simulink model "kinematic_model"  (R2022b)
settings: Solver=FixedStepAuto  StartTime=0.0  StopTime=24  FixedStep=0.1  RelTol=1e-3
settings Model: Creator=Rajgir  LastModifiedBy=rajgir
settings DebuggingCC: UnconnectedInputMsg=warning  UnconnectedOutputMsg=warning  UnconnectedLineMsg=warning
settings ModelReferenceCC: EnableRefExpFcnMdlSchedulingChecks=on
settings RTWCC: DLArmComputeVersion=19.05

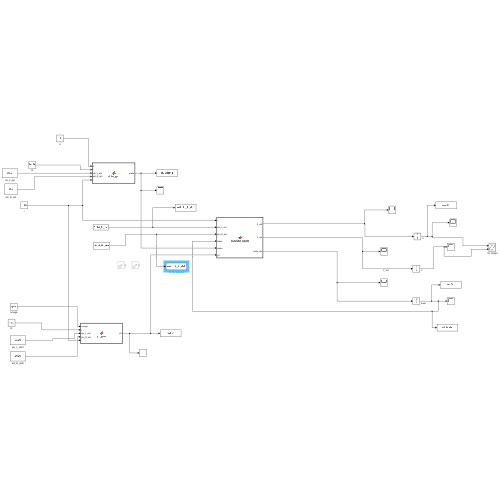
[thumbnail: Simulink's stored preview of the top-level diagram]
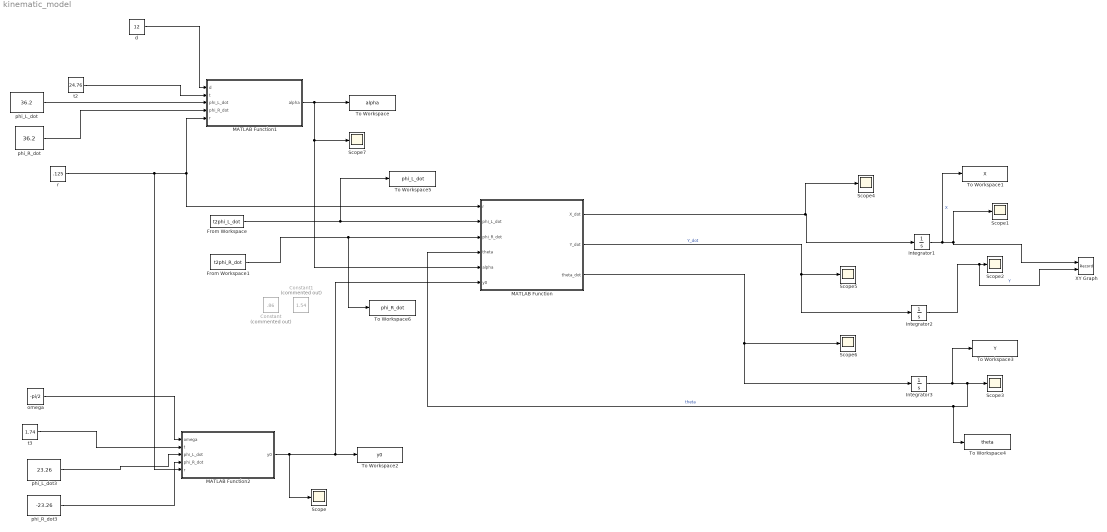
== system kinematic_model ==
  Constant : Constant  Commented=on  Value=.86
  Constant1 : Constant  Commented=on  Value=1.54
  From Workspace : FromWorkspace  VariableName=t2phi_L_dot  SampleTime=.1
  From Workspace1 : FromWorkspace  VariableName=t2phi_R_dot  SampleTime=.1
  Integrator1 : Integrator
  Integrator2 : Integrator
  Integrator3 : Integrator  InitialCondition=pi/2
  MATLAB Function : MATLAB Function  TreatAsAtomicUnit=on
  MATLAB Function1 : MATLAB Function  TreatAsAtomicUnit=on
  MATLAB Function2 : MATLAB Function  TreatAsAtomicUnit=on
  Scope{,1..7} (8 alike) : Scope
  To Workspace : ToWorkspace  VariableName=alpha  SampleTime=-1
  To Workspace1 : ToWorkspace  VariableName=X  SampleTime=-1
  To Workspace2 : ToWorkspace  VariableName=y0  SampleTime=-1
  To Workspace3 : ToWorkspace  VariableName=Y  SampleTime=-1
  To Workspace4 : ToWorkspace  VariableName=theta  SampleTime=-1
  To Workspace5 : ToWorkspace  VariableName=phi_L_dot  SampleTime=-1
  To Workspace6 : ToWorkspace  VariableName=phi_R_dot  SampleTime=-1
  XY Graph : Record  FileSettingsInternal="{\"entries\":[{\"content\":{\"excelSettings\":{\"content\":{},\"type\":\"Streamout.ExcelSettings\"}},\"type\":\"Streamout.FileSettingStorage\",\"uuid\":\"74dff1ba-9ac4-49e6-a5a9-d9f2a2d52b08\"}],\"packageUris\":[\"http://schema.mathworks.com/mf0/streamout_blocks/R2020a\"],\"version\":\"1.0\"}"  Layout=[1 1]  SignalsInternal="{\"entries\":[{\"content\":{\"signals\":[{\"content\":{\"blockPath\":[\"kinem_4WDD_hom_p_test_workspace/XY Graph\"],\"channel\":[],\"dimensions\":[1],\"domain\":\"kinem_4WDD_hom_p_test_workspace/XY Graph\",\"lineColor\":\"#a2142f\",\"plots\":[1],\"port\":1,\"sid\":[\"\"],\"signalID\":19,\"signalName\":\"X\"},\"type\":\"RecordBlkView.Signal\",\"uuid\":\"0c54e238-fd94-41af-aab3-b701ba149f00\"},{\"content\":{\"blockPath\":[\"kinem_4WDD_hom_p_test_workspace/XY Graph\"],\"channel\":[],\"dimensions\":[1],\"domain\":\"kinem_4WDD_hom_p_test_workspace/XY Graph\",\"lineColor\":\"#139fff\",\"plots\":[1],\"port\":2,\"sid\":[\"\"],\"signalID\":23,\"signalName\":\"Y\"},\"type\":\"RecordBlkView.Signal\",\"uuid\":\"0df5b6cb-212d-4097-94d9-53b1708521eb\"}]},\"type\":\"RecordBlkView.InputSignals\",\"uuid\":\"4189ed81-e381-4474-ba4b-bd6d2c2501e0\"}],\"packageUris\":[\"http://schema.mathworks.com/mf0/streamout_blocks/R2020a\"],\"version\":\"1.0\"}"  VisualizationBindings="{\"xyplotplugin\":{\"info\":[{\"series\":[{\"bindingParametersList\":[{\"parameter\":\"X-Axis\",\"signalID\":19,\"signalName\":\"X\"},{\"parameter\":\"Y-Axis\",\"signalID\":23,\"signalName\":\"Y\"}],\"seriesID\":41180}],\"subplotID\":1}]}}"  CompatibilityTag=XY  st=-1
  d : Constant  Value=12  SampleTime=0
  omega : Constant  Value=-pi/2
  phi_L_dot : Constant  Value=36.2  SampleTime=0
  phi_L_dot3 : Constant  Value=23.26  SampleTime=0
  phi_R_dot : Constant  Value=36.2  SampleTime=0
  phi_R_dot3 : Constant  Value=-23.26  SampleTime=0
  r : Constant  Value=.125  OutMax=3  SampleTime=0
  t2 : Constant  Value=24.76
  t3 : Constant  Value=1.74
  wires:
  MATLAB Function/1(X_dot) -> Scope4/1, Integrator1/1
  MATLAB Function/2(Y_dot) -> Integrator2/1, Scope5/1  "Y_dot"
  Integrator1/1 -> To Workspace1/1, XY Graph/1, Scope1/1  "X"
  Integrator2/1 -> XY Graph/2, Scope2/1  "Y"
  Integrator3/1 -> To Workspace3/1, To Workspace4/1, MATLAB Function/4(theta), Scope3/1  "theta"
  MATLAB Function/3(theta_dot) -> Integrator3/1, Scope6/1
  r/1 -> MATLAB Function1/5(r), MATLAB Function/1(r), MATLAB Function2/5(r)
  MATLAB Function1/1(alpha) -> To Workspace/1, MATLAB Function/5(alpha), Scope7/1
  MATLAB Function2/1(y0) -> MATLAB Function/6(y0), To Workspace2/1, Scope/1
  phi_L_dot/1 -> MATLAB Function1/3(phi_L_dot)
  phi_R_dot/1 -> MATLAB Function1/4(phi_R_dot)
  d/1 -> MATLAB Function1/1(d)
  t2/1 -> MATLAB Function1/2(t)
  phi_L_dot3/1 -> MATLAB Function2/3(phi_L_dot)
  phi_R_dot3/1 -> MATLAB Function2/4(phi_R_dot)
  t3/1 -> MATLAB Function2/2(t)
  omega/1 -> MATLAB Function2/1(omega)
  From Workspace/1 -> To Workspace5/1, MATLAB Function/2(phi_L_dot)
  From Workspace1/1 -> To Workspace6/1, MATLAB Function/3(phi_R_dot)

== matlab function kinematic_model/MATLAB Function1 ==
  data: d input; alpha output; t input; phi_L_dot input; phi_R_dot input; r input
function alpha  = alpha_gen(d, t,  phi_L_dot,  phi_R_dot, r)

phi_L_dot_rad= phi_L_dot*2*pi/60;  phi_R_dot_rad= phi_R_dot*2*pi/60;

alpha = 2*d / (((phi_R_dot_rad + phi_L_dot_rad))*(t*r));



end

== matlab function kinematic_model/MATLAB Function ==
  data: r input; phi_L_dot input; X_dot output; phi_R_dot input; theta input; Y_dot output; theta_dot output; alpha input; y0 input
function [X_dot, Y_dot, theta_dot] = kinematic_model(r, phi_L_dot, phi_R_dot, theta, alpha, y0)

    phi_L_dot_rad= phi_L_dot*2*pi/60;  phi_R_dot_rad= phi_R_dot*2*pi/60;
    
    X_dot = (r * alpha .* phi_L_dot_rad / 2) .* cos(theta) + (r * alpha .* phi_R_dot_rad / 2) .* cos(theta);
    
    Y_dot = (r * alpha .* phi_L_dot_rad / 2) .* sin(theta) + (r * alpha .* phi_R_dot_rad / 2) .* sin(theta);
    
    theta_dot = -(r * alpha .* phi_L_dot_rad / (2 * y0)) + (r * alpha .* phi_R_dot_rad / (2 * y0));

end

== matlab function kinematic_model/MATLAB Function2 ==
  data: omega input; y0 output; t input; phi_L_dot input; phi_R_dot input; r input
function y0  = y0_gen(omega, t,  phi_L_dot,  phi_R_dot, r)


phi_L_dot_rad= phi_L_dot*2*pi/60;  phi_R_dot_rad= phi_R_dot*2*pi/60;


y0 = ((phi_R_dot_rad * r - phi_L_dot_rad)* r)*t / (2 * omega);





end
